simulink model "Logan"  (R2024b)
settings: Solver=ode4  StartTime=0  StopTime=inf  FixedStep=0.01  RelTol=1e-3
values from neighbouring files (symbols this model uses):
  AltPoint = 100000    [Logan_init.m]
  area_secao = 79.402*1.5    (= 119.103)    [Logan_init.m]
  b = 9    [Logan_init.m]
  c = 15.252    [Logan_init.m]
  cp = 1003    [Logan_init.m]
  E = 110e9    (= 110000000000)    [Logan_init.m]
  eta_comb = 0.95    [Logan_init.m]
  Fuel_Freeze = 0    [Logan_init.m]
  g = 9.80665    [Logan_init.m]
  gamma = 1.4    [Logan_init.m]
  GammaRef_deg = 0    [Logan_init.m]
  h1 = 0.5746    [Logan_init.m]
  h2 = 0.7752    [Logan_init.m]
  h3 = 0.1502    [Logan_init.m]
  hc = h1 + h2 + h3    (= 1.5)    [Logan_init.m]
  he = 2.6    [Logan_init.m]
  Inertia = [Ixx 0 -Ixz; 0 Iyy 0; -Ixz 0 Izz]    [Logan_init.m]
  L = 22.5    [Logan_init.m]
  L_inlet = 5.5    [Logan_init.m]
  La = 5    [Logan_init.m]
  LHV = 120 * 10^6    (= 120000000)    [Logan_init.m]
  Ln0 = 4.8    [Logan_init.m]
  MachPoint = 10    [Logan_init.m]
  Manual_Control = 0    [Logan_init.m]
  MW_air = 28.85    [Logan_init.m]
  MW_H2 = 2.00    (= 2)    [Logan_init.m]
  PA_EngineMode = 0    [Logan_init.m]
  PA_LatMode = 2    [Logan_init.m]
  PA_LongMode = 2    [Logan_init.m]
  PA_TECSEngineInput = 0    [Logan_init.m]
  PhiPoint = 0    [Logan_init.m]
  R = 287    [Logan_init.m]
  RefMass_kg = 31000    [Logan_init.m]
  S = 91.5    [Logan_init.m]
  tau1 = 3.1    [Logan_init.m]
  tau2 = 18.23    [Logan_init.m]
  TECS_ON = 0    [Logan_init.m]
  theta1 = 4    [Logan_init.m]
  theta2 = 6    [Logan_init.m]
  theta_n = 4    [Logan_init.m]
  ThetaPoint = 0    [Logan_init.m]
  Trimming = 0    [Logan_init.m]    (also in Logan_trim.m)
  w = 3.000    (= 3)    [Logan_init.m]
  Waypoint_idx = 1    [Logan_init.m]
  Waypoints = [ ... (first row only)    [Logan_init.m]
  x_a = 3.7    [Logan_init.m]
  x_inlet = 6    [Logan_init.m]
  x_n0 = 3    [Logan_init.m]
  xf_m = 0    [Logan_init.m]
  y_cg = 0    [Logan_init.m]
  z_a = 0.4    [Logan_init.m]
  z_cg = -0.996    [Logan_init.m]
  z_inlet = 0.7    [Logan_init.m]
  zf_m = 0    [Logan_init.m]
undefined symbols (not defined in the file or in its folder): Earth, Receive, Send, WGS84
libraries: simulink x4, spsFirstOrderFilterLib x4, aerolibactuator x3, aerolibfltsims x2, aerolibatmos2 x1, aerolibtransform2 x1, aerolibanimutils x1, dspswit3 x1, spsEdgeDetectorLib x1
(part 3 of 5)

== matlab function Logan/Aero/MATLAB Function1 ==
  data: M input; b input; CL output; Alpha_deg input; Beta input; R_elev input; L_elev input; L_Rud input; R_Rud input; c input; CD output; p input; q input; r input; TAS input; CY output; Cll output; Cm output; Cn output
function [CL, CD, CY, Cll, Cm, Cn] = fcn(M, b, Alpha_deg, Beta, R_elev, L_elev, L_Rud, R_Rud, c, p, q, r, TAS)

% scale_factor_span = 6 / 18.288;
% scale_factor_area = 91.51 / 334.73;
% scale_factor_chord = 15.252 / 24.384;
% scale_factor_elevon = 3.13/28.133;
% scale_factor_rudder = 1.136/49.07;

scale_factor_span = 1;
scale_factor_area = 1;
scale_factor_chord = 1;
scale_factor_elevon = 1;
scale_factor_rudder = 1;

%CD

    CDbv = (+ 8.717E-02 - 3.307E-02*M + 3.179E-03*Alpha_deg ...
        - 1.250E-04*(Alpha_deg*M) + 5.036E-03*M^2 ...
        - 1.100E-03*Alpha_deg^2 + 1.405E-07*(Alpha_deg*M)^2 ...
        - 3.658E-04*M^3 + 3.175E-04*Alpha_deg^3 + 1.274E-05*M^4 ...
        -2.985E-05*Alpha_deg^4 - 1.705E-07 *M^5 + 9.766E-07*Alpha_deg^5)*scale_factor_area;

    CD_R_elev = (+ 1*(4.5548e-004) + Alpha_deg.*(2.5411e-005) + M.*(-1.1436e-004) ...
        + R_elev.*(-3.6417e-005) + ((Alpha_deg.*M).*R_elev).*( -5.3015e-007) ...
        + (Alpha_deg.^2).*( 3.2187e-006) + (M.^2).*(3.0140e-006) ...
        + (R_elev.^2).*(6.9629e-006) ...
        + (((Alpha_deg.*M).*R_elev).^2).*(2.1026e-012))*scale_factor_elevon;

    CD_L_elev = (+ 1*(4.5548e-004) + Alpha_deg.*(2.5411e-005) + M.*(-1.1436e-004) ...
        + L_elev.*(-3.6417e-005) + ((Alpha_deg.*M).*L_elev).*( -5.3015e-007) ...
        + (Alpha_deg.^2).*( 3.2187e-006) + (M.^2).*(3.0140e-006) ...
        + (L_elev.^2).*(6.9629e-006) ...
        + (((Alpha_deg.*M).*L_elev).^2).*(2.1026e-012))*scale_factor_elevon;

    CD_R_Rud= ((+ 7.50E-04 - 2.29E-05*Alpha_deg - 9.69E-05*M - 1.83E-06*R_Rud ...
        + 9.13E-09*(Alpha_deg*M)*R_Rud + 8.76E-07*Alpha_deg^2 ...
        + 2.70E-06*M^2 + 1.97E-06*R_Rud^2 - 1.77E-11*((Alpha_deg*M)*R_Rud)^2)/2)*scale_factor_rudder;

    CD_L_Rud= ((+ 7.50E-04 - 2.29E-05*Alpha_deg - 9.69E-05*M - 1.83E-06*L_Rud ...
        + 9.13E-09*(Alpha_deg*M)*L_Rud + 8.76E-07*Alpha_deg^2 ...
        + 2.70E-06*M^2 + 1.97E-06*L_Rud^2 - 1.77E-11*((Alpha_deg*M)*L_Rud)^2)/2)*scale_factor_rudder;

    CD = CDbv + CD_R_elev + CD_L_elev + CD_L_Rud +CD_R_Rud;

    %CL

    CLbv = (- 8.19E-02 + 4.70E-02*M + 1.86E-02*Alpha_deg ...
        - 4.73E-04*(Alpha_deg*M) - 9.19E-03*M^2 - 1.52E-04*Alpha_deg^2 ...
        + 5.99E-07*(Alpha_deg*M)^2 + 7.74E-04*M^3 ...
        + 4.08E-06 *Alpha_deg^3 - 2.93E-05*M^4 - 3.91E-07*Alpha_deg^4 ...
        + 4.12E-07*M^5 + 1.30E-08*Alpha_deg^5)*scale_factor_area;

    CL_R_elev = (- 1.45E-05 + 1.01E-04*Alpha_deg + 7.10E-06 *M - 4.14E-04*R_elev ...
        - 3.51E-06 *(Alpha_deg*R_elev) + 4.70E-06*(Alpha_deg*M) ...
        + 8.72E-06*(M*R_elev) - 1.70E-07*(Alpha_deg*M)*R_elev)*scale_factor_elevon;

    CL_L_elev = (- 1.45E-05 + 1.01E-04*Alpha_deg + 7.10E-06 *M - 4.14E-04*L_elev ...
        - 3.51E-06 *(Alpha_deg*L_elev) + 4.70E-06*(Alpha_deg*M) ...
        + 8.72E-06*(M*L_elev) - 1.70E-07*(Alpha_deg*M)*L_elev)*scale_factor_elevon ;

    CL = CLbv + CL_L_elev + CL_R_elev;

    %CY

    CYB = ((0) + M* (-2.9253e-001) + Alpha_deg.*(2.8803e-003) ...
        + (Alpha_deg.*M).* (-2.8943e-004) + (M.^2).*(5.4822e-002) ...
        + (Alpha_deg.^2).* (7.3535e-004) ...
        + ((Alpha_deg.*M.^2).^2).* (-4.6490e-009) ...
        + (((Alpha_deg.^2).*M).^2).*(-2.0675e-008) ...
        + ((Alpha_deg.*M).^2).*(4.6205e-006) ...
        + (((Alpha_deg.^2).* M.^2).^2).*(2.6144e-011) ...
        + (M.^3).*(-4.3203e-003) ...
        + (Alpha_deg.^3).*(-3.7405e-004) + (M.^4).*(1.5495e-004) ...
        + (Alpha_deg.^4).*(2.8183e-005) + (M.^5).*(-2.0829e-006) ...
        + (Alpha_deg.^5).* (-5.2083e-007))*scale_factor_area ;

    CY_R_elev = (- 1.02E-06 - 1.12E-07*Alpha_deg + 4.48E-07*M + 2.27E-07*R_elev ...
        + 4.11E-09 *(Alpha_deg*M)*R_elev + 2.82E-09*Alpha_deg^2 ...
        - 2.36E-08*M^2 - 5.04E-08*R_elev^2 ...
        + 4.50E-14*((Alpha_deg*M)*R_elev)^2)*scale_factor_elevon;

    CY_L_elev = (-(- 1.02E-06 - 1.12E-07*Alpha_deg + 4.48E-07*M + 2.27E-07*L_elev ...
        + 4.11E-09 *(Alpha_deg*M)*L_elev + 2.82E-09*Alpha_deg^2 ...
        - 2.36E-08*M^2 ...
        - 5.04E-08*L_elev^2 + 4.50E-14*((Alpha_deg*M)*L_elev)^2))*scale_factor_elevon;

    CY_R_Rud= scale_factor_rudder*(- 1.43E-18 + 4.86E-20*Alpha_deg+ 1.86E-19*M + 3.84E-04*R_Rud ...
        - 1.17E-05*(Alpha_deg*R_Rud) - 1.07E-05*(M*R_Rud) ...
        + 2.60E-07*(Alpha_deg*M)*R_Rud)/2;

    CY_L_Rud= scale_factor_rudder*(- 1.43E-18 + 4.86E-20*Alpha_deg+ 1.86E-19*M + 3.84E-04*L_Rud ...
        - 1.17E-05*(Alpha_deg*L_Rud) - 1.07E-05*(M*L_Rud) ...
        + 2.60E-07*(Alpha_deg*M)*L_Rud)/2;

     CY = CYB*Beta + CY_L_elev +CY_R_elev +CY_L_Rud +CY_R_Rud;

    %Cll

    Cllbv = (- 1.402E-01 + 3.326E-02*M - 7.590E-04*Alpha_deg ...
        + 8.596E-06*(Alpha_deg*M) - 3.794E-03*M^2 ...
        + 2.354E-06*Alpha_deg^2 -1.044E-08*(Alpha_deg*M)^2 ...
        + 2.219E-04*M^3 - 8.964E-18*Alpha_deg^3 - 6.462E-06*M^4 ...
        + 3.803E-19*Alpha_deg^4 + 7.419E-08*M^5 -3.353E-21*Alpha_deg^5)*scale_factor_span;

    Cll_R_elev= (+ 3.570E-04 - 9.569E-05*Alpha_deg - 3.598E-05*M + 1.170E-04*R_elev ...
        + 2.794E-08*(Alpha_deg*M)*R_elev + 4.950E-06*Alpha_deg^2 ...
        + 1.411E-06*M^2 - 1.160E-06*R_elev^2 ...
        - 4.641E-11*((Alpha_deg*M)*R_elev)^2)*scale_factor_elevon;

    Cll_L_elev= (-(3.570E-04 - 9.569E-05*Alpha_deg - 3.598E-05*M + 1.170E-04*L_elev ...
        + 2.794E-08*(Alpha_deg*M)*L_elev + 4.950E-06*Alpha_deg^2 ...
        + 1.411E-06*M^2 - 1.160E-06*L_elev^2 ...
        - 4.641E-11*((Alpha_deg*M)*L_elev)^2))*scale_factor_elevon;

    Cll_R_Rud=scale_factor_rudder*(- 5.0103E-19 + 6.2723E-20*Alpha_deg + 2.3418E-20*M ...
        + 0.00011441*R_Rud - 2.6824E-06*(Alpha_deg*R_Rud) ...
        - 3.4201E-21*(Alpha_deg*M) - 3.5496E-06*(M*R_Rud) ...
        + 5.5547E-08*(Alpha_deg*M)*R_Rud)/2;

    Cll_L_Rud=scale_factor_rudder*(- 5.0103E-19 + 6.2723E-20*Alpha_deg + 2.3418E-20*M ...
        + 0.00011441*L_Rud - 2.6824E-06*(Alpha_deg*L_Rud) ...
        - 3.4201E-21*(Alpha_deg*M) - 3.5496E-06*(M*L_Rud) ...
        + 5.5547E-08*(Alpha_deg*M)*L_Rud)/2;

    Cllr = + 3.82E-01 - 1.06E-01*M + 1.94E-03* Alpha_deg ...
        - 8.15E-05*(Alpha_deg*M) + 1.45E-02*M^2 - 9.76E-06*Alpha_deg^2 ...
        + 4.49E-08*(Alpha_deg*M)^2 - 1.02E-03*M^3 ...
        - 2.70E-07*Alpha_deg^3 + 3.56E-05*M^4 + 3.19E-08*Alpha_deg^4 ...
        - 4.81E-07*M^5 -1.06E-09*Alpha_deg^5;

    Cllp = - 2.99E-01 + 7.47E-02*M + 1.38E-03*Alpha_deg ...
        - 8.78E-05*(Alpha_deg*M) - 9.13E-03*M^2 - 2.04E-04*Alpha_deg^2 ...
        - 1.52E-07*(Alpha_deg*M)^2 + 5.73E-04*M^3 ...
        - 3.86E-05*Alpha_deg^3 - 1.79E-05*M^4 + 4.21E-06*Alpha_deg^4 ...
        + 2.20E-07*M^5 - 1.15E-07*Alpha_deg^5;

    Cll = Cllbv*Beta + Cll_L_elev + Cll_R_elev + Cll_L_Rud + Cll_R_Rud + Cllr*((r*b)/(2*TAS)) + Cllp*((p*b)/(2*TAS));

    %Cm

    Cmbv = (- 2.192E-02 + 7.739E-03*M - 2.260E-03*Alpha_deg ...
        + 1.808E-04*(Alpha_deg*M) - 8.849E-04*M^2 ...
        + 2.616E-04*Alpha_deg^2 -2.880E-07*(Alpha_deg*M)^2 ...
        + 4.617E-05*M^3 -7.887E-05*Alpha_deg^3 -1.143E-06*M^4 ...
        + 8.288E-06*Alpha_deg^4 + 1.082E-08*M^5 - 2.789E-07*Alpha_deg^5)*scale_factor_chord;

    Cm_R_elev = (- 5.67E-05 - 6.59E-05*Alpha_deg -1.51E-06*M + 2.89E-04*R_elev ...
        + 4.48E-06*(Alpha_deg*R_elev) - 4.46E-06*(Alpha_deg*M) ...
        - 5.87E-06*(M*R_elev) ...
        + 9.72E-08*(Alpha_deg*M)*R_elev)*scale_factor_elevon;

    Cm_L_elev = (- 5.67E-05 - 6.59E-05*Alpha_deg -1.51E-06*M + 2.89E-04*L_elev ...
        + 4.48E-06*(Alpha_deg*L_elev) - 4.46E-06*(Alpha_deg*M) ...
        - 5.87E-06*(M*L_elev) ...
        + 9.72E-08*(Alpha_deg*M)*L_elev)*scale_factor_elevon;

    Cm_R_Rud= scale_factor_rudder*(- 2.79E-05*Alpha_deg - 5.89E-08*(Alpha_deg)^2 + 1.58E-03*(M)^2 ...
        + 6.42E-08*(Alpha_deg)^3 - 6.69E-04*(M)^3 - 2.10E-08*(Alpha_deg)^4 ...
        + 1.05E-04*(M)^4 + 1.43E-07*(R_Rud)^4 + 3.14E-09*(Alpha_deg)^5 ...
        - 7.74E-06*(M)^5 - 4.77E-22*(R_Rud)^5 - 2.18E-10*(Alpha_deg)^6 ...
        + 2.70E-07*(M)^6 - 3.38E-10*(R_Rud)^6 + 5.74E-12*(Alpha_deg)^7 ...
        - 3.58E-09*(M)^7 + 2.63E-24*(R_Rud)^7)/2;

    Cm_L_Rud= scale_factor_rudder*(- 2.79E-05*Alpha_deg - 5.89E-08*(Alpha_deg)^2 + 1.58E-03*(M)^2 ...
        + 6.42E-08*(Alpha_deg)^3 - 6.69E-04*(M)^3 - 2.10E-08*(Alpha_deg)^4 ...
        + 1.05E-04*(M)^4 + 1.43E-07*(L_Rud)^4 + 3.14E-09*(Alpha_deg)^5 ...
        - 7.74E-06*(M)^5 - 4.77E-22*(L_Rud)^5 - 2.18E-10*(Alpha_deg)^6 ...
        + 2.70E-07*(M)^6 - 3.38E-10*(L_Rud)^6 + 5.74E-12*(Alpha_deg)^7 ...
        - 3.58E-09*(M)^7 + 2.63E-24*(L_Rud)^7)/2;

    Cm_q = - 1.36E+00 + 3.86E-01*M + 7.85E-04*Alpha_deg ...
        + 1.40E-04*(Alpha_deg*M) - 5.42E-02 *M^2 ...
        + 2.36E-03*Alpha_deg^2 - 1.95E-06 *(Alpha_deg*M)^2 ...
        + 3.80E-03*M^3 - 1.48E-03 *Alpha_deg^3 - 1.30E-04 *M^4 ...
        + 1.69E-04*Alpha_deg^4 + 1.71E-06*M^5 - 5.93E-06 *Alpha_deg^5;

    Cm = (Cmbv + Cm_L_elev + Cm_R_elev + Cm_L_Rud + Cm_R_Rud + Cm_q*((q*c)/(2*TAS)));

    %Cn

    Cnbv = (+ (0) + Alpha_deg.* (6.9980e-004) +M.*(5.9115e-002) ...
        + (Alpha_deg.*M).*(-7.5250e-005) + ((Alpha_deg).^2).*(2.5160e-004) ...
        + ((M).^2).*(-1.4824e-002) ...
        + ((Alpha_deg.*M).^2).*(-2.1924e-007) ...
        + ((Alpha_deg).^3).*(-1.0777e-004) + ((M).^3).*(1.2692e-003) ...
        + ((Alpha_deg.*M).^3).* (1.0707e-008) ...
        + ((Alpha_deg).^4).*(9.4989e-006) + ((M).^4).*(-4.7098e-005) ...
        + ((Alpha_deg.*M).^4).*(-5.5472e-011) ...
        + ((Alpha_deg).^5).* (-2.5953e-007)+ ((M).^5).*(6.4284e-007) ...
        + ((Alpha_deg.*M).^5).* (8.5863e-014))*scale_factor_span;

    Cn_R_elev = (+ 2.10E-04 + 1.83E-05*Alpha_deg - 3.56E-05*M - 1.30E-05*R_elev ...
        - 8.93E-08*(Alpha_deg*M)*R_elev -6.39E-07*Alpha_deg^2 + 8.16E-07*M^2 ...
        + 1.97E-06*R_elev^2 + 1.41E-11*((Alpha_deg*M)*R_elev)^2)*scale_factor_elevon;

    Cn_L_elev = (-(2.10E-04 + 1.83E-05*Alpha_deg - 3.56E-05*M - 1.30E-05*L_elev ...
        - 8.93E-08*(Alpha_deg*M)*L_elev -6.39E-07*Alpha_deg^2 + 8.16E-07*M^2 ...
        + 1.97E-06*L_elev^2 + 1.41E-11*((Alpha_deg*M)*L_elev)^2))*scale_factor_elevon;

    Cn_R_Rud= scale_factor_rudder*(+ 2.85E-18 - 3.59E-19 *Alpha_deg -1.26E-19*M -5.28E-04*R_Rud ...
        + 1.39E-05*(Alpha_deg*R_Rud) + 1.57E-20*(Alpha_deg*M) ...
        + 1.65E-05*(M*R_Rud) ...
        - 3.13E-07*(Alpha_deg*M)*R_Rud)/2;

    Cn_L_Rud= scale_factor_rudder*(+ 2.85E-18 - 3.59E-19 *Alpha_deg -1.26E-19*M -5.28E-04*L_Rud ...
        + 1.39E-05*(Alpha_deg*L_Rud) + 1.57E-20*(Alpha_deg*M) ...
        + 1.65E-05*(M*L_Rud) ...
        - 3.13E-07*(Alpha_deg*M)*L_Rud)/2;

    Cnp = + 3.68E-01 -9.79E-02*M + 7.61E-16*Alpha_deg + 1.24E-02*M^2 ...
        - 4.64E-16*Alpha_deg^2 -8.05E-04*M^3 +1.01E-16*Alpha_deg^3 ...
        + 2.57E-05*M^4 ...
        - 9.18E-18*Alpha_deg^4 -3.20E-07* M^5 + 2.96E-19*Alpha_deg^5;

    Cnr = - 2.41E+00 + 5.96E-01*M - 2.74E-03*Alpha_deg ...
        + 2.09E-04*(Alpha_deg*M) - 7.57E-02*M^2 ...
        + 1.15E-03* Alpha_deg^2 - 6.53E-08*(Alpha_deg*M)^2 ...
        + 4.90E-03*M^3 - 3.87E-04*Alpha_deg^3 - 1.57E-04*M^4 ...
        + 3.60E-05*Alpha_deg^4 + 1.96E-06*M^5 - 1.18E-06*Alpha_deg^5;

    Cn = Cnbv*Beta + Cn_L_elev + Cn_R_elev + Cn_L_Rud + Cn_R_Rud + Cnr*((r*b)/(2*TAS)) + Cnp*((p*b)/(2*TAS));

end

== matlab function Logan/Estructural ==
  data: F input; deformation output; A input; E input; L input; m input; freq_n output; Delta_tau_f output
function [deformation, freq_n, Delta_tau_f] = calcEstrutura(F, A, E, L, m)
% CALCESTRUTURA - Calcula a deformação, frequência natural e ângulo resultante
% 
% Entradas:
%   F  - Força aplicada (N)
%   A  - Área da seção transversal (m²)
%   E  - Módulo de elasticidade (Pa)
%   L  - Comprimento da estrutura (m)
%   m  - Massa da estrutura (kg)
%
% Saídas:
%   deformacao - Deformação elástica total da estrutura (m)
%   freq_natural - Frequência natural da estrutura (rad/s)
%   angulo - Ângulo resultante da deformação (graus)

    % Tensão aplicada
    sigma = F / A;
    
    % Deformação unitária (adimensional)
    epsilon = sigma / E;
    
    % Deformação total
    deformation = epsilon * L;
    
    % Rigidez estrutural
    k = (E * A) / L;
    
    % Frequência natural (rad/s)
    freq_n = sqrt(k / m);
    
    % Ângulo resultante da deformação (em graus)
    Delta_tau_f = atan(deformation / L) * (180 / pi);
end

== matlab function Logan/Outer Loop/HeadingMode/MATLAB Function ==
  data: lat input; heading_ref output; lon input; waypoints input; waypoint_idx input; psi_atual input; psi_corrigido output; erro output; tol_dist input; next_waypoint_idx output; dist_to_wp output
function [heading_ref, psi_corrigido, erro, next_waypoint_idx, dist_to_wp] = calculateHeadingWaypoints(lat, lon, waypoints, waypoint_idx, psi_atual, tol_dist)
% CALCULATEHEADINGWAYPOINTS - Calcula o heading de referência para um conjunto de waypoints.
% Garante a troca de waypoints quando o avião atinge o atual dentro da tolerância.
    
    % **1. Verificar Índices Válidos**
    num_waypoints = size(waypoints, 1); % Número total de waypoints
    if waypoint_idx > num_waypoints
        waypoint_idx = num_waypoints; % Fixa no último waypoint
    elseif waypoint_idx < 1
        waypoint_idx = 1; % Garante que o índice seja válido
    end

    % **2. Extrair Waypoint Atual**
    lat_wp = waypoints(waypoint_idx, 1); % Latitude do waypoint atual
    lon_wp = waypoints(waypoint_idx, 2); % Longitude do waypoint atual

    % **3. Calcular Distância ao Waypoint Atual**
    R = 6371000; % Raio médio da Terra em metros
    lat_rad = deg2rad(lat);
    lon_rad = deg2rad(lon);
    lat_wp_rad = deg2rad(lat_wp);
    lon_wp_rad = deg2rad(lon_wp);

    % Fórmula de Haversine para calcular a distância
    delta_lat = lat_wp_rad - lat_rad;
    delta_lon = lon_wp_rad - lon_rad;
    a = sin(delta_lat / 2)^2 + cos(lat_rad) * cos(lat_wp_rad) * sin(delta_lon / 2)^2;
    c = 2 * atan2(sqrt(a), sqrt(1 - a));
    dist_to_wp = R * c; % Distância ao waypoint atual em metros

    % **4. Trocar Waypoint se Dentro da Tolerância**
    if dist_to_wp < tol_dist
        if waypoint_idx < num_waypoints
            waypoint_idx = waypoint_idx + 1; % Avança para o próximo waypoint
        end
    end

    % **5. Atualizar Waypoint Atual**
    lat_wp = waypoints(waypoint_idx, 1); % Atualizar latitude do waypoint atual
    lon_wp = waypoints(waypoint_idx, 2); % Atualizar longitude do waypoint atual

    % **6. Calcular Heading para o Waypoint Atual**
    delta_lon = lon_wp_rad - lon_rad;
    x = sin(delta_lon) * cos(lat_wp_rad);
    y = cos(lat_rad) * sin(lat_wp_rad) - sin(lat_rad) * cos(lat_wp_rad) * cos(delta_lon);
    heading_base = rad2deg(atan2(x, y));

    % Normalizar o heading para [0, 360)
    heading_ref = mod(heading_base + 360, 360);

    % **7. Ajustar o Psi Atual**

    % Normalizar o heading atual para [0, 360)
    psi_corrigido = mod(psi_atual + 360, 360);

    % **8. Calcular o Erro Angular**

    % Calcular o erro angular bruto
    erro_bruto = heading_ref - psi_corrigido;

    % Normalizar o erro para [-180, 180]
    erro = mod(erro_bruto + 180, 360) - 180;

    % **9. Retornar Índice do Próximo Waypoint**
    next_waypoint_idx = waypoint_idx;
end
